simulink model "csv_planning"  (R2023a)
settings: configuration reference "config" (kept outside this file)
settings Model: DataDictionary=model_config.sldd  Creator=huangcheng  LastModifiedBy=Administrator
settings ConfigSetRef: SourceName=config

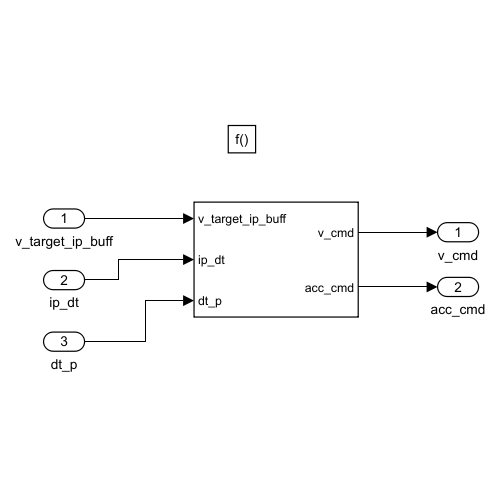
[thumbnail: Simulink's stored preview of the top-level diagram]
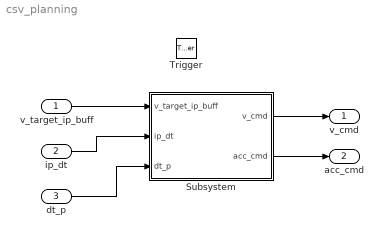
== system csv_planning ==
  v_target_ip_buff : Inport  OutDataTypeStr=single  PortDimensions=4
  ip_dt : Inport  Port=2
  dt_p : Inport  Port=3
  Trigger : TriggerPort  TriggerType=function-call  VariantControl=(inherit)  PortDimensions=1
  Subsystem : Subsystem
  v_cmd : Outport
  acc_cmd : Outport  Port=2
  wires:
  dt_p/1 -> Subsystem/3(dt_p)
  v_target_ip_buff/1 -> Subsystem/1(v_target_ip_buff)
  ip_dt/1 -> Subsystem/2(ip_dt)
  Subsystem/1(v_cmd) -> v_cmd/1
  Subsystem/2(acc_cmd) -> acc_cmd/1

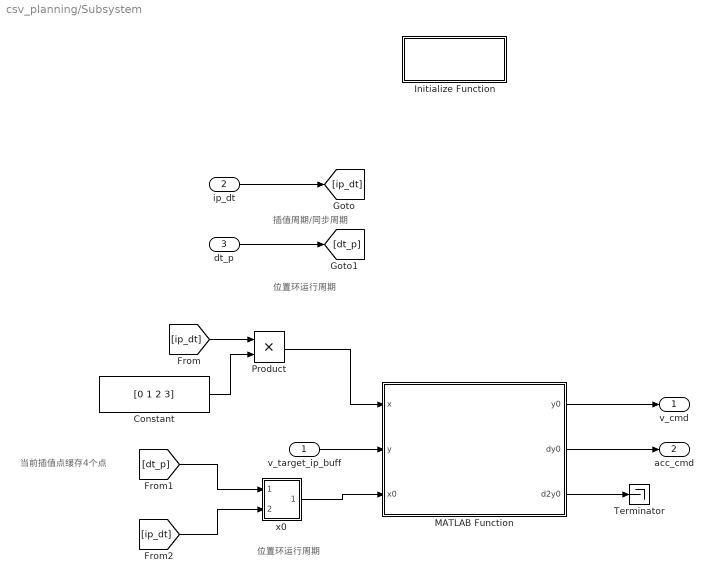
== system csv_planning/Subsystem ==
  note: 插值周期/同步周期
  note: 当前插值点缓存4个点
  note: 位置环运行周期
  note: 位置环运行周期
  v_target_ip_buff : Inport  OutDataTypeStr=single  PortDimensions=4
  ip_dt : Inport  Port=2
  dt_p : Inport  Port=3
  Constant : Constant  Value=[0 1 2 3]  OutDataTypeStr=single
  Initialize Function : Subsystem  TreatAsAtomicUnit=on
  MATLAB Function : MATLAB Function  SystemSampleTime=10e-5
  Product : Product
  Terminator : Terminator
  x0 : Subsystem
  v_cmd : Outport
  acc_cmd : Outport  Port=2
  wires:
  MATLAB Function/3(d2y0) -> Terminator/1
  MATLAB Function/2(dy0) -> acc_cmd/1
  Product/1 -> MATLAB Function/1(x)
  ip_dt/1 -> [ip_dt]
  Constant/1 -> Product/2
  [ip_dt] -> Product/1
  x0/1(Out1) -> MATLAB Function/3(x0)
  [dt_p] -> x0/1(In1)
  dt_p/1 -> [dt_p]
  [ip_dt] -> x0/2(In2)
  MATLAB Function/1(y0) -> v_cmd/1
  v_target_ip_buff/1 -> MATLAB Function/2(y)

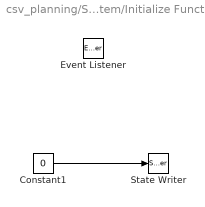
== system csv_planning/Subsystem/Initialize Function ==
  Constant1 : Constant  Value=0  OutDataTypeStr=boolean
  Event Listener : EventListener  DisableCoverage=on  EventName=reset
  State Writer : StateWriter  StateOwnerBlock=../../x0/Delay  StateName=x0_init_flag
  wires:
  Constant1/1 -> State Writer/1

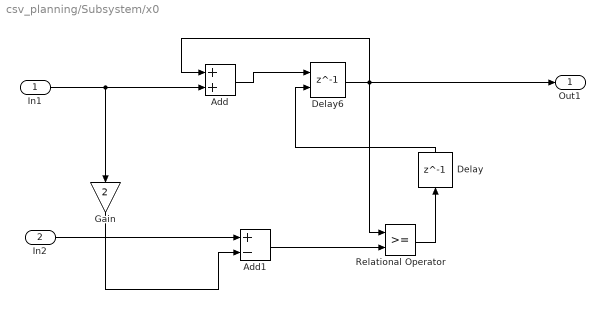
== system csv_planning/Subsystem/x0 ==
  In1 : Inport
  In2 : Inport  Port=2
  Add : Sum
  Add1 : Sum  Inputs=+-
  Delay : Delay  DelayLength=1  StateName=x0_init_flag
  Delay6 : Delay  DelayLength=1  ExternalReset=Rising  StateName=x0_now
      settings: InputPortMap=u0,r5
  Gain : Gain  Gain=2
  Relational Operator : RelationalOperator  OutDataTypeStr=boolean  RndMeth=Simplest  InputSameDT=off
  Out1 : Outport
  wires:
  Delay/1 -> Delay6/2
  In2/1 -> Add1/1
  In1/1 -> Gain/1, Add/2
  Relational Operator/1 -> Delay/1
  Add1/1 -> Relational Operator/2
  Gain/1 -> Add1/2
  Delay6/1 -> Out1/1, Add/1, Relational Operator/1
  Add/1 -> Delay6/1

== matlab function csv_planning/Subsystem/MATLAB Function ==
  data: x input; y input; y0 output; x0 input; dy0 output; d2y0 output
function [y0, dy0, d2y0]  = interpolateSignal(x,y,x0)
 
 % 可选插值方法pchip、 makima 、spline一阶导数和二阶导数
    % 输入:
    %   pp - 返回的分段多项式结构
    %   x0 - 要计算的点（可以是向量）
    % 输出:
    %   y0  - 函数值
    %   dy0 - 一阶导数
    %   d2y0 - 二阶导数

    % 提取分段插值起点, 插值计算都减去起点
    y_init = y(1);
    yy = y - y_init;

    pp = makima(x, yy);


    % 1. 计算函数值
    y0 = ppval(pp, x0) + y_init;
    
     % 方法二：手动从系数计算
    breaks = pp.breaks;
    coefs = pp.coefs;

    %x0必须始终在插值第一段

    c = coefs(1, :);  % 系数为 [a, b, c, d]，对应 (x-break)^3, (x-break)^2, (x-break)^1, 常数项
    t = x0 - breaks(1);
    % 一阶导数
    dy0 = 3*c(1)*t^2 + 2*c(2)*t + c(3);
    % 二阶导数
    d2y0 = 6*c(1)*t + 2*c(2);

end
